simulink model "speedgoat_test_SN5659_R2021b"  (R2021b)
settings: Solver=FixedStepDiscrete  StartTime=0.0  StopTime=inf  RelTol=1e-3
PreLoadFcn:
  | Ts_IO107 = 0.001;
  | Ts_IO107 = 0.001;
  | Ts_IO133 = 0.001
  | 
  | Ts_IO204 = 0.001;
  | 
  | 
  | Ts_IO503 = 0.01;
  | 
  | ts_IO612 = 1e-3;
  | Ts_IO682 = 0.005;
  | Ts_IO941 = 0.01;
InitFcn:
  | Ts_IO107 = 0.001;
  | Ts_IO107 = 0.001;
  | Ts_IO133 = 0.001
  | 
  | Ts_IO204 = 0.001;
  | 
  | 
  | Ts_IO503 = 0.01;
  | 
  | ts_IO612 = 1e-3;
  | Ts_IO682 = 0.005;
  | Ts_IO941 = 0.01;
StopFcn:
  | if isfile(['sdi_view_',bdroot,'.mldatx'])
  |  Simulink.sdi.clearPreferences();
  |  Simulink.sdi.view();
  |  pause(3);
  |  Simulink.sdi.loadView(['sdi_view_',bdroot,]);
  | end
undefined symbols (not defined in the file): C, IO682, standard
libraries: speedgoatlib_IO682 x161, simulink x49, slrealtimeseriallib x16, canmsglib x12, speedgoatlib_serial x9, speedgoatlib_IO612 x9, speedgoatlib_IO133 x5, speedgoatlib_IO107 x4, speedgoatlib_IO204 x3, speedgoatlib_IO421 x3, speedgoatlib_PIL x1
(part 3 of 4)

== system speedgoat_test_SN5659_R2021b/IO682/Encode Channel 3 ==
  Constant : Constant  Value=150.159  SampleTime=Ts_IO682
  Counter Limited : simulink/Sources/Counter Limited  uplimit=300  tsamp=Ts_IO682
  Data Type Conversion : DataTypeConversion
  Encode 1 : speedgoatlib_IO682/Encode v2   parMode=Message Sequence  parLabel=100  parDataType=[1]  parResolution=[1024]  parBits=[10]  parSdi=[2]  parSsm=[3]  parCustomDataType=Raw  parDataLSB=9  parDataMSB=31  parBitPosition=[9, 31]  parScaleBNR=1  parExponent=8  parMantissa=14  parEnSSM=off
      settings: SourceProductName=Simulink Real-Time: Speedgoat I/O Blockset
  Encode 2 : speedgoatlib_IO682/Encode v2   parMode=Message Sequence  parLabel=101  parDataType=[2]  parResolution=[.1]  parBits=[0]  parSdi=[2]  parSsm=[0]  parCustomDataType=Raw  parDataLSB=9  parDataMSB=31  parBitPosition=[9, 31]  parScaleBNR=1  parExponent=8  parMantissa=14  parEnSSM=off
      settings: SourceProductName=Simulink Real-Time: Speedgoat I/O Blockset
  Encode 3 : speedgoatlib_IO682/Encode v2   parMode=Message Sequence  parLabel=102  parDataType=[1]  parResolution=[65536]  parBits=[16]  parSdi=[2]  parSsm=[3]  parCustomDataType=Raw  parDataLSB=9  parDataMSB=31  parBitPosition=[9, 31]  parScaleBNR=1  parExponent=8  parMantissa=14  parEnSSM=off
      settings: SourceProductName=Simulink Real-Time: Speedgoat I/O Blockset
  Encode 4 : speedgoatlib_IO682/Encode v2   parMode=Message Sequence  parLabel=103  parDataType=[0]  parResolution=[1]  parBits=[0]  parSdi=[0]  parSsm=[0]  parCustomDataType=Raw  parDataLSB=9  parDataMSB=31  parBitPosition=[9, 31]  parScaleBNR=1  parExponent=8  parMantissa=14  parEnSSM=off
      settings: SourceProductName=Simulink Real-Time: Speedgoat I/O Blockset
  Mux1 : Mux
  Prepare RAW value : Subsystem
  Random number : RandomNumber  Mean=150  Variance=10  SampleTime=Ts_IO682
  Sine wave : Sin  Amplitude=10000  Bias=13000  Frequency=2*pi*0.01  SampleTime=Ts_IO682
  Out1 : Outport
  wires:
  Encode 4/1 -> Mux1/4
  Mux1/1 -> Out1/1
  Counter Limited/1 -> Data Type Conversion/1
  Sine wave/1 -> Encode 3/1
  Encode 3/1 -> Mux1/3
  Encode 1/1 -> Mux1/1
  Random number/1 -> Encode 1/1
  Encode 2/1 -> Mux1/2
  Prepare RAW value/1(Out1) -> Encode 4/1
  Constant/1 -> Prepare RAW value/1(In1)
  Data Type Conversion/1 -> Encode 2/1

== system speedgoat_test_SN5659_R2021b/IO682/Encode Channel 4 ==
  Constant : Constant  Value=200.159  SampleTime=Ts_IO682
  Counter Limited : simulink/Sources/Counter Limited  uplimit=400  tsamp=Ts_IO682
  Data Type Conversion : DataTypeConversion
  Encode 1 : speedgoatlib_IO682/Encode v2   parMode=Message Sequence  parLabel=100  parDataType=[1]  parResolution=[1024]  parBits=[10]  parSdi=[2]  parSsm=[3]  parCustomDataType=Raw  parDataLSB=9  parDataMSB=31  parBitPosition=[9, 31]  parScaleBNR=1  parExponent=8  parMantissa=14  parEnSSM=off
      settings: SourceProductName=Simulink Real-Time: Speedgoat I/O Blockset
  Encode 2 : speedgoatlib_IO682/Encode v2   parMode=Message Sequence  parLabel=101  parDataType=[2]  parResolution=[.1]  parBits=[0]  parSdi=[2]  parSsm=[0]  parCustomDataType=Raw  parDataLSB=9  parDataMSB=31  parBitPosition=[9, 31]  parScaleBNR=1  parExponent=8  parMantissa=14  parEnSSM=off
      settings: SourceProductName=Simulink Real-Time: Speedgoat I/O Blockset
  Encode 3 : speedgoatlib_IO682/Encode v2   parMode=Message Sequence  parLabel=102  parDataType=[1]  parResolution=[65536]  parBits=[16]  parSdi=[2]  parSsm=[3]  parCustomDataType=Raw  parDataLSB=9  parDataMSB=31  parBitPosition=[9, 31]  parScaleBNR=1  parExponent=8  parMantissa=14  parEnSSM=off
      settings: SourceProductName=Simulink Real-Time: Speedgoat I/O Blockset
  Encode 4 : speedgoatlib_IO682/Encode v2   parMode=Message Sequence  parLabel=103  parDataType=[0]  parResolution=[1]  parBits=[0]  parSdi=[0]  parSsm=[0]  parCustomDataType=Raw  parDataLSB=9  parDataMSB=31  parBitPosition=[9, 31]  parScaleBNR=1  parExponent=8  parMantissa=14  parEnSSM=off
      settings: SourceProductName=Simulink Real-Time: Speedgoat I/O Blockset
  Mux1 : Mux
  Prepare RAW value : Subsystem
  Random number : RandomNumber  Mean=200  Variance=10  SampleTime=Ts_IO682
  Sine wave : Sin  Amplitude=10000  Bias=14000  Frequency=2*pi*0.01  SampleTime=Ts_IO682
  Out1 : Outport
  wires:
  Encode 4/1 -> Mux1/4
  Mux1/1 -> Out1/1
  Counter Limited/1 -> Data Type Conversion/1
  Sine wave/1 -> Encode 3/1
  Encode 3/1 -> Mux1/3
  Encode 1/1 -> Mux1/1
  Random number/1 -> Encode 1/1
  Encode 2/1 -> Mux1/2
  Prepare RAW value/1(Out1) -> Encode 4/1
  Constant/1 -> Prepare RAW value/1(In1)
  Data Type Conversion/1 -> Encode 2/1

== system speedgoat_test_SN5659_R2021b/IO682/Encode Channel 5 ==
  note: Encode block definitions:
      | 1. Label 100, BNR, Scale 1024, 10 bits, SDI 2, SSM 3
      | 2. Label 101, BCD, Resolution 0.1, SDI 2, SSM from sign of input
      | 3. Label 102, BNR, Scale 65536, 16 bits, SDI 2, SSM 3
      | 4. Label 103, RAW, Resolution/Scale, SDI and SSM aren't taken
      |         from the Encode block mask, but leave placeholders in the arrays.
      |         These values are inserted into the RAW value in the Prepare
      |         RAW value subsystem.  Label is also inserted manually.
  Constant : Constant  Value=250.159  SampleTime=Ts_IO682
  Counter Limited : simulink/Sources/Counter Limited  uplimit=500  tsamp=Ts_IO682
  Data Type Conversion : DataTypeConversion
  Encode 1 : speedgoatlib_IO682/Encode v2   parMode=Message Sequence  parLabel=100  parDataType=[1]  parResolution=[1024]  parBits=[10]  parSdi=[2]  parSsm=[3]  parCustomDataType=Raw  parDataLSB=9  parDataMSB=31  parBitPosition=[9, 31]  parScaleBNR=1  parExponent=8  parMantissa=14  parEnSSM=off
      settings: SourceProductName=Simulink Real-Time: Speedgoat I/O Blockset
  Encode 2 : speedgoatlib_IO682/Encode v2   parMode=Message Sequence  parLabel=103  parDataType=[0]  parResolution=[1024]  parBits=[0]  parSdi=[0]  parSsm=[0]  parCustomDataType=Raw  parDataLSB=9  parDataMSB=31  parBitPosition=[9, 31]  parScaleBNR=1  parExponent=8  parMantissa=14  parEnSSM=off
      settings: SourceProductName=Simulink Real-Time: Speedgoat I/O Blockset
  Encode 3 : speedgoatlib_IO682/Encode v2   parMode=Message Sequence  parLabel=102  parDataType=[1]  parResolution=[65536]  parBits=[16]  parSdi=[2]  parSsm=[3]  parCustomDataType=Raw  parDataLSB=9  parDataMSB=31  parBitPosition=[9, 31]  parScaleBNR=1  parExponent=8  parMantissa=14  parEnSSM=off
      settings: SourceProductName=Simulink Real-Time: Speedgoat I/O Blockset
  Encode 5 : speedgoatlib_IO682/Encode v2   parMode=Message Sequence  parLabel=101  parDataType=[2]  parResolution=[.1]  parBits=[0]  parSdi=[2]  parSsm=[0]  parCustomDataType=Raw  parDataLSB=9  parDataMSB=31  parBitPosition=[9, 31]  parScaleBNR=1  parExponent=8  parMantissa=14  parEnSSM=off
      settings: SourceProductName=Simulink Real-Time: Speedgoat I/O Blockset
  Mux : Mux
  Prepare RAW value : Subsystem
  Random number : RandomNumber  Mean=250  Variance=10  SampleTime=Ts_IO682
  Sine wave : Sin  Amplitude=10000  Bias=15000  Frequency=2*pi*0.01  SampleTime=Ts_IO682
  Out1 : Outport
  wires:
  Mux/1 -> Out1/1
  Sine wave/1 -> Encode 3/1
  Encode 2/1 -> Mux/4
  Encode 3/1 -> Mux/3
  Encode 5/1 -> Mux/2
  Random number/1 -> Encode 1/1
  Encode 1/1 -> Mux/1
  Counter Limited/1 -> Data Type Conversion/1
  Prepare RAW value/1(Out1) -> Encode 2/1
  Constant/1 -> Prepare RAW value/1(In1)
  Data Type Conversion/1 -> Encode 5/1

== system speedgoat_test_SN5659_R2021b/IO682/Encode Channel 6 ==
  Constant : Constant  Value=300.159  SampleTime=Ts_IO682
  Counter Limited : simulink/Sources/Counter Limited  uplimit=600  tsamp=Ts_IO682
  Data Type Conversion : DataTypeConversion
  Encode 1 : speedgoatlib_IO682/Encode v2   parMode=Message Sequence  parLabel=100  parDataType=[1]  parResolution=[1024]  parBits=[10]  parSdi=[2]  parSsm=[3]  parCustomDataType=Raw  parDataLSB=9  parDataMSB=31  parBitPosition=[9, 31]  parScaleBNR=1  parExponent=8  parMantissa=14  parEnSSM=off
      settings: SourceProductName=Simulink Real-Time: Speedgoat I/O Blockset
  Encode 2 : speedgoatlib_IO682/Encode v2   parMode=Message Sequence  parLabel=101  parDataType=[2]  parResolution=[.1]  parBits=[0]  parSdi=[2]  parSsm=[0]  parCustomDataType=Raw  parDataLSB=9  parDataMSB=31  parBitPosition=[9, 31]  parScaleBNR=1  parExponent=8  parMantissa=14  parEnSSM=off
      settings: SourceProductName=Simulink Real-Time: Speedgoat I/O Blockset
  Encode 3 : speedgoatlib_IO682/Encode v2   parMode=Message Sequence  parLabel=102  parDataType=[1]  parResolution=[65536]  parBits=[16]  parSdi=[2]  parSsm=[3]  parCustomDataType=Raw  parDataLSB=9  parDataMSB=31  parBitPosition=[9, 31]  parScaleBNR=1  parExponent=8  parMantissa=14  parEnSSM=off
      settings: SourceProductName=Simulink Real-Time: Speedgoat I/O Blockset
  Encode 4 : speedgoatlib_IO682/Encode v2   parMode=Message Sequence  parLabel=103  parDataType=[0]  parResolution=[1]  parBits=[0]  parSdi=[0]  parSsm=[0]  parCustomDataType=Raw  parDataLSB=9  parDataMSB=31  parBitPosition=[9, 31]  parScaleBNR=1  parExponent=8  parMantissa=14  parEnSSM=off
      settings: SourceProductName=Simulink Real-Time: Speedgoat I/O Blockset
  Mux1 : Mux
  Prepare RAW value : Subsystem
  Random number : RandomNumber  Mean=300  Variance=10  SampleTime=Ts_IO682
  Sine wave : Sin  Amplitude=10000  Bias=16000  Frequency=2*pi*0.01  SampleTime=Ts_IO682
  Out1 : Outport
  wires:
  Encode 2/1 -> Mux1/2
  Prepare RAW value/1(Out1) -> Encode 4/1
  Encode 3/1 -> Mux1/3
  Encode 1/1 -> Mux1/1
  Constant/1 -> Prepare RAW value/1(In1)
  Sine wave/1 -> Encode 3/1
  Random number/1 -> Encode 1/1
  Mux1/1 -> Out1/1
  Counter Limited/1 -> Data Type Conversion/1
  Encode 4/1 -> Mux1/4
  Data Type Conversion/1 -> Encode 2/1

== system speedgoat_test_SN5659_R2021b/IO682/Encode Channel 7 ==
  Constant : Constant  Value=350.159  SampleTime=Ts_IO682
  Counter Limited : simulink/Sources/Counter Limited  uplimit=700  tsamp=Ts_IO682
  Data Type Conversion : DataTypeConversion
  Encode 1 : speedgoatlib_IO682/Encode v2   parMode=Message Sequence  parLabel=100  parDataType=[1]  parResolution=[1024]  parBits=[10]  parSdi=[2]  parSsm=[3]  parCustomDataType=Raw  parDataLSB=9  parDataMSB=31  parBitPosition=[9, 31]  parScaleBNR=1  parExponent=8  parMantissa=14  parEnSSM=off
      settings: SourceProductName=Simulink Real-Time: Speedgoat I/O Blockset
  Encode 2 : speedgoatlib_IO682/Encode v2   parMode=Message Sequence  parLabel=101  parDataType=[2]  parResolution=[.1]  parBits=[0]  parSdi=[2]  parSsm=[0]  parCustomDataType=Raw  parDataLSB=9  parDataMSB=31  parBitPosition=[9, 31]  parScaleBNR=1  parExponent=8  parMantissa=14  parEnSSM=off
      settings: SourceProductName=Simulink Real-Time: Speedgoat I/O Blockset
  Encode 3 : speedgoatlib_IO682/Encode v2   parMode=Message Sequence  parLabel=102  parDataType=[1]  parResolution=[65536]  parBits=[16]  parSdi=[2]  parSsm=[3]  parCustomDataType=Raw  parDataLSB=9  parDataMSB=31  parBitPosition=[9, 31]  parScaleBNR=1  parExponent=8  parMantissa=14  parEnSSM=off
      settings: SourceProductName=Simulink Real-Time: Speedgoat I/O Blockset
  Encode 4 : speedgoatlib_IO682/Encode v2   parMode=Message Sequence  parLabel=103  parDataType=[0]  parResolution=[1]  parBits=[0]  parSdi=[0]  parSsm=[0]  parCustomDataType=Raw  parDataLSB=9  parDataMSB=31  parBitPosition=[9, 31]  parScaleBNR=1  parExponent=8  parMantissa=14  parEnSSM=off
      settings: SourceProductName=Simulink Real-Time: Speedgoat I/O Blockset
  Mux1 : Mux
  Prepare RAW value : Subsystem
  Random number : RandomNumber  Mean=350  Variance=10  SampleTime=Ts_IO682
  Sine wave : Sin  Amplitude=10000  Bias=17000  Frequency=2*pi*0.01  SampleTime=Ts_IO682
  Out1 : Outport
  wires:
  Encode 4/1 -> Mux1/4
  Mux1/1 -> Out1/1
  Counter Limited/1 -> Data Type Conversion/1
  Sine wave/1 -> Encode 3/1
  Encode 3/1 -> Mux1/3
  Encode 1/1 -> Mux1/1
  Random number/1 -> Encode 1/1
  Encode 2/1 -> Mux1/2
  Prepare RAW value/1(Out1) -> Encode 4/1
  Constant/1 -> Prepare RAW value/1(In1)
  Data Type Conversion/1 -> Encode 2/1

== system speedgoat_test_SN5659_R2021b/IO682/Encode Channel 8 ==
  Constant : Constant  Value=400.159  SampleTime=Ts_IO682
  Counter Limited : simulink/Sources/Counter Limited  uplimit=800  tsamp=Ts_IO682
  Data Type Conversion : DataTypeConversion
  Encode 1 : speedgoatlib_IO682/Encode v2   parMode=Message Sequence  parLabel=100  parDataType=[1]  parResolution=[1024]  parBits=[10]  parSdi=[2]  parSsm=[3]  parCustomDataType=Raw  parDataLSB=9  parDataMSB=31  parBitPosition=[9, 31]  parScaleBNR=1  parExponent=8  parMantissa=14  parEnSSM=off
      settings: SourceProductName=Simulink Real-Time: Speedgoat I/O Blockset
  Encode 2 : speedgoatlib_IO682/Encode v2   parMode=Message Sequence  parLabel=101  parDataType=[2]  parResolution=[.1]  parBits=[0]  parSdi=[2]  parSsm=[0]  parCustomDataType=Raw  parDataLSB=9  parDataMSB=31  parBitPosition=[9, 31]  parScaleBNR=1  parExponent=8  parMantissa=14  parEnSSM=off
      settings: SourceProductName=Simulink Real-Time: Speedgoat I/O Blockset
  Encode 3 : speedgoatlib_IO682/Encode v2   parMode=Message Sequence  parLabel=102  parDataType=[1]  parResolution=[65536]  parBits=[16]  parSdi=[2]  parSsm=[3]  parCustomDataType=Raw  parDataLSB=9  parDataMSB=31  parBitPosition=[9, 31]  parScaleBNR=1  parExponent=8  parMantissa=14  parEnSSM=off
      settings: SourceProductName=Simulink Real-Time: Speedgoat I/O Blockset
  Encode 4 : speedgoatlib_IO682/Encode v2   parMode=Message Sequence  parLabel=103  parDataType=[0]  parResolution=[1]  parBits=[0]  parSdi=[0]  parSsm=[0]  parCustomDataType=Raw  parDataLSB=9  parDataMSB=31  parBitPosition=[9, 31]  parScaleBNR=1  parExponent=8  parMantissa=14  parEnSSM=off
      settings: SourceProductName=Simulink Real-Time: Speedgoat I/O Blockset
  Mux1 : Mux
  Prepare RAW value : Subsystem
  Random number : RandomNumber  Mean=400  Variance=10  SampleTime=Ts_IO682
  Sine wave : Sin  Amplitude=10000  Bias=18000  Frequency=2*pi*0.01  SampleTime=Ts_IO682
  Out1 : Outport
  wires:
  Encode 4/1 -> Mux1/4
  Mux1/1 -> Out1/1
  Counter Limited/1 -> Data Type Conversion/1
  Sine wave/1 -> Encode 3/1
  Encode 3/1 -> Mux1/3
  Encode 1/1 -> Mux1/1
  Random number/1 -> Encode 1/1
  Encode 2/1 -> Mux1/2
  Prepare RAW value/1(Out1) -> Encode 4/1
  Constant/1 -> Prepare RAW value/1(In1)
  Data Type Conversion/1 -> Encode 2/1

== system speedgoat_test_SN5659_R2021b/IO682/Encode Channel 9 ==
  note: Encode block definitions:
      | 1. Label 100, BNR, Scale 1024, 10 bits, SDI 2, SSM 3
      | 2. Label 101, BCD, Resolution 0.1, SDI 2, SSM from sign of input
      | 3. Label 102, BNR, Scale 65536, 16 bits, SDI 2, SSM 3
      | 4. Label 103, RAW, Resolution/Scale, SDI and SSM aren't taken
      |         from the Encode block mask, but leave placeholders in the arrays.
      |         These values are inserted into the RAW value in the Prepare
      |         RAW value subsystem.  Label is also inserted manually.
  Constant : Constant  Value=450.159  SampleTime=Ts_IO682
  Counter Limited : simulink/Sources/Counter Limited  uplimit=900  tsamp=Ts_IO682
  Data Type Conversion : DataTypeConversion
  Encode 1 : speedgoatlib_IO682/Encode v2   parMode=Message Sequence  parLabel=100  parDataType=[1]  parResolution=[1024]  parBits=[10]  parSdi=[2]  parSsm=[3]  parCustomDataType=Raw  parDataLSB=9  parDataMSB=31  parBitPosition=[9, 31]  parScaleBNR=1  parExponent=8  parMantissa=14  parEnSSM=off
      settings: SourceProductName=Simulink Real-Time: Speedgoat I/O Blockset
  Encode 2 : speedgoatlib_IO682/Encode v2   parMode=Message Sequence  parLabel=103  parDataType=[0]  parResolution=[1024]  parBits=[0]  parSdi=[0]  parSsm=[0]  parCustomDataType=Raw  parDataLSB=9  parDataMSB=31  parBitPosition=[9, 31]  parScaleBNR=1  parExponent=8  parMantissa=14  parEnSSM=off
      settings: SourceProductName=Simulink Real-Time: Speedgoat I/O Blockset
  Encode 3 : speedgoatlib_IO682/Encode v2   parMode=Message Sequence  parLabel=102  parDataType=[1]  parResolution=[65536]  parBits=[16]  parSdi=[2]  parSsm=[3]  parCustomDataType=Raw  parDataLSB=9  parDataMSB=31  parBitPosition=[9, 31]  parScaleBNR=1  parExponent=8  parMantissa=14  parEnSSM=off
      settings: SourceProductName=Simulink Real-Time: Speedgoat I/O Blockset
  Encode 5 : speedgoatlib_IO682/Encode v2   parMode=Message Sequence  parLabel=101  parDataType=[2]  parResolution=[.1]  parBits=[0]  parSdi=[2]  parSsm=[0]  parCustomDataType=Raw  parDataLSB=9  parDataMSB=31  parBitPosition=[9, 31]  parScaleBNR=1  parExponent=8  parMantissa=14  parEnSSM=off
      settings: SourceProductName=Simulink Real-Time: Speedgoat I/O Blockset
  Mux : Mux
  Prepare RAW value : Subsystem
  Random number : RandomNumber  Mean=450  Variance=10  SampleTime=Ts_IO682
  Sine wave : Sin  Amplitude=10000  Bias=19000  Frequency=2*pi*0.01  SampleTime=Ts_IO682
  Out1 : Outport
  wires:
  Mux/1 -> Out1/1
  Sine wave/1 -> Encode 3/1
  Encode 2/1 -> Mux/4
  Encode 3/1 -> Mux/3
  Encode 5/1 -> Mux/2
  Random number/1 -> Encode 1/1
  Encode 1/1 -> Mux/1
  Counter Limited/1 -> Data Type Conversion/1
  Prepare RAW value/1(Out1) -> Encode 2/1
  Constant/1 -> Prepare RAW value/1(In1)
  Data Type Conversion/1 -> Encode 5/1

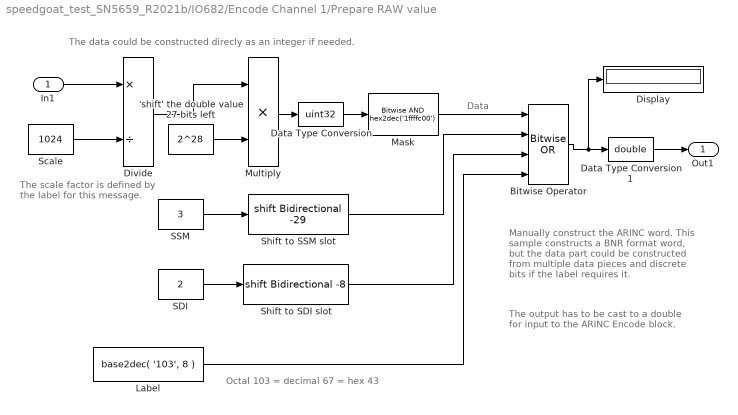
== system speedgoat_test_SN5659_R2021b/IO682/Encode Channel 1/Prepare RAW value ==
  note: The scale factor is
      | defined by the label
      | for this message.
  note: Manually construct the ARINC word.
      | This sample constructs a BNR format
      | word, but the data part could be
      | constructed from multiple data pieces
      | and discrete bits if the label requires it.
  note: Data
  note: The output has to be cast to a double
      | for input to the ARINC Encode block.
  note: The data could be constructed direcly as an integer if needed.
  note: Octal 103 = decimal 67 = hex 43
  In1 : Inport
  'shift' the double value 27 bits left : Constant  Value=2^28  OutDataTypeStr=double
  Bitwise Operator : simulink/Logic and Bit Operations/Bitwise Operator  logicop=OR  UseBitMask=off  NumInputPorts=4  BitMask=bin2dec('11011001')  BitMaskRealWorld=Stored Integer
  Data Type Conversion : DataTypeConversion  OutDataTypeStr=uint32
  Data Type Conversion1 : DataTypeConversion  OutDataTypeStr=double
  Display : Display
      settings: Format=hex (Stored Integer)
  Divide : Product  Inputs=*/
  Label : Constant  Value=base2dec( '103', 8 )  OutDataTypeStr=uint32
  "Mask " : simulink/Logic and Bit Operations/Bitwise Operator  logicop=AND  UseBitMask=on  BitMask=hex2dec('1ffffc00')  BitMaskRealWorld=Stored Integer
  Multiply : Product  Inputs=**
  SDI : Constant  Value=2  OutDataTypeStr=uint32
  SSM : Constant  Value=3  OutDataTypeStr=uint32
  Scale : Constant  Value=1024  OutDataTypeStr=double
  Shift to SDI slot : ArithShift  BitShiftNumber=-8
  Shift to SSM slot : ArithShift  BitShiftNumber=-29
  Out1 : Outport
  wires:
  In1/1 -> Divide/1
  Scale/1 -> Divide/2
  'shift' the double value 27 bits left/1 -> Multiply/2
  Divide/1 -> Multiply/1
  Multiply/1 -> Data Type Conversion/1
  Data Type Conversion/1 -> "Mask "/1
  "Mask "/1 -> Bitwise Operator/1
  SSM/1 -> Shift to SSM slot/1
  SDI/1 -> Shift to SDI slot/1
  Shift to SSM slot/1 -> Bitwise Operator/2
  Shift to SDI slot/1 -> Bitwise Operator/3
  Label/1 -> Bitwise Operator/4
  Bitwise Operator/1 -> Data Type Conversion1/1, Display/1
  Data Type Conversion1/1 -> Out1/1

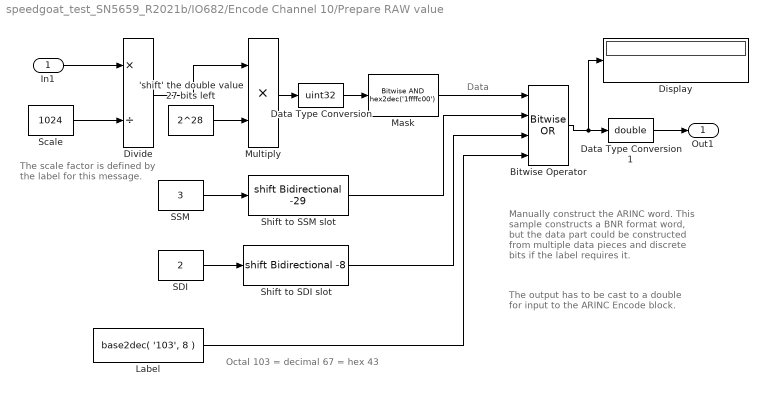
== system speedgoat_test_SN5659_R2021b/IO682/Encode Channel 10/Prepare RAW value ==
  note: Octal 103 = decimal 67 = hex 43
  note: The output has to be cast to a double
      | for input to the ARINC Encode block.
  note: Data
  note: Manually construct the ARINC word.
      | This sample constructs a BNR format
      | word, but the data part could be
      | constructed from multiple data pieces
      | and discrete bits if the label requires it.
  note: The scale factor is
      | defined by the label
      | for this message.
  In1 : Inport
  'shift' the double value 27 bits left : Constant  Value=2^28  OutDataTypeStr=double
  Bitwise Operator : simulink/Logic and Bit Operations/Bitwise Operator  logicop=OR  UseBitMask=off  NumInputPorts=4  BitMask=bin2dec('11011001')  BitMaskRealWorld=Stored Integer
  Data Type Conversion : DataTypeConversion  OutDataTypeStr=uint32
  Data Type Conversion1 : DataTypeConversion  OutDataTypeStr=double
  Display : Display
      settings: Format=hex (Stored Integer)
  Divide : Product  Inputs=*/
  Label : Constant  Value=base2dec( '103', 8 )  OutDataTypeStr=uint32
  "Mask " : simulink/Logic and Bit Operations/Bitwise Operator  logicop=AND  UseBitMask=on  BitMask=hex2dec('1ffffc00')  BitMaskRealWorld=Stored Integer
  Multiply : Product  Inputs=**
  SDI : Constant  Value=2  OutDataTypeStr=uint32
  SSM : Constant  Value=3  OutDataTypeStr=uint32
  Scale : Constant  Value=1024  OutDataTypeStr=double
  Shift to SDI slot : ArithShift  BitShiftNumber=-8
  Shift to SSM slot : ArithShift  BitShiftNumber=-29
  Out1 : Outport
  wires:
  Data Type Conversion1/1 -> Out1/1
  Bitwise Operator/1 -> Display/1, Data Type Conversion1/1
  Label/1 -> Bitwise Operator/4
  Shift to SDI slot/1 -> Bitwise Operator/3
  Shift to SSM slot/1 -> Bitwise Operator/2
  SDI/1 -> Shift to SDI slot/1
  SSM/1 -> Shift to SSM slot/1
  "Mask "/1 -> Bitwise Operator/1
  Data Type Conversion/1 -> "Mask "/1
  Multiply/1 -> Data Type Conversion/1
  Divide/1 -> Multiply/1
  'shift' the double value 27 bits left/1 -> Multiply/2
  Scale/1 -> Divide/2
  In1/1 -> Divide/1

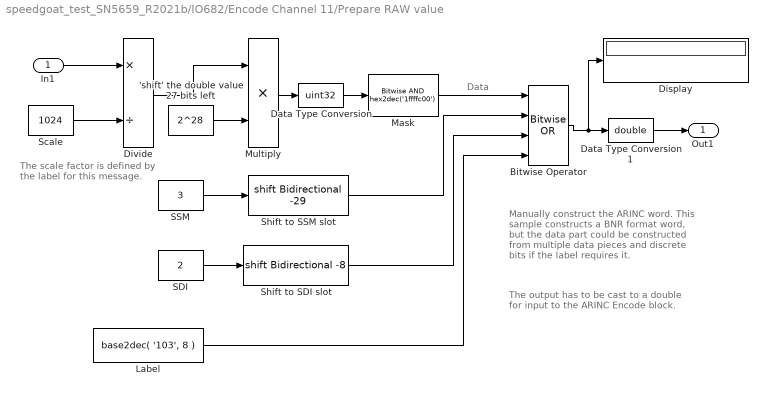
== system speedgoat_test_SN5659_R2021b/IO682/Encode Channel 11/Prepare RAW value ==
  note: The scale factor is
      | defined by the label
      | for this message.
  note: Manually construct the ARINC word.
      | This sample constructs a BNR format
      | word, but the data part could be
      | constructed from multiple data pieces
      | and discrete bits if the label requires it.
  note: Data
  note: The output has to be cast to a double
      | for input to the ARINC Encode block.
  In1 : Inport
  'shift' the double value 27 bits left : Constant  Value=2^28  OutDataTypeStr=double
  Bitwise Operator : simulink/Logic and Bit Operations/Bitwise Operator  logicop=OR  UseBitMask=off  NumInputPorts=4  BitMask=bin2dec('11011001')  BitMaskRealWorld=Stored Integer
  Data Type Conversion : DataTypeConversion  OutDataTypeStr=uint32
  Data Type Conversion1 : DataTypeConversion  OutDataTypeStr=double
  Display : Display
      settings: Format=hex (Stored Integer)
  Divide : Product  Inputs=*/
  Label : Constant  Value=base2dec( '103', 8 )  OutDataTypeStr=uint32
  "Mask " : simulink/Logic and Bit Operations/Bitwise Operator  logicop=AND  UseBitMask=on  BitMask=hex2dec('1ffffc00')  BitMaskRealWorld=Stored Integer
  Multiply : Product  Inputs=**
  SDI : Constant  Value=2  OutDataTypeStr=uint32
  SSM : Constant  Value=3  OutDataTypeStr=uint32
  Scale : Constant  Value=1024  OutDataTypeStr=double
  Shift to SDI slot : ArithShift  BitShiftNumber=-8
  Shift to SSM slot : ArithShift  BitShiftNumber=-29
  Out1 : Outport
  wires:
  In1/1 -> Divide/1
  Scale/1 -> Divide/2
  'shift' the double value 27 bits left/1 -> Multiply/2
  Divide/1 -> Multiply/1
  Multiply/1 -> Data Type Conversion/1
  Data Type Conversion/1 -> "Mask "/1
  "Mask "/1 -> Bitwise Operator/1
  SSM/1 -> Shift to SSM slot/1
  SDI/1 -> Shift to SDI slot/1
  Shift to SSM slot/1 -> Bitwise Operator/2
  Shift to SDI slot/1 -> Bitwise Operator/3
  Label/1 -> Bitwise Operator/4
  Bitwise Operator/1 -> Data Type Conversion1/1, Display/1
  Data Type Conversion1/1 -> Out1/1

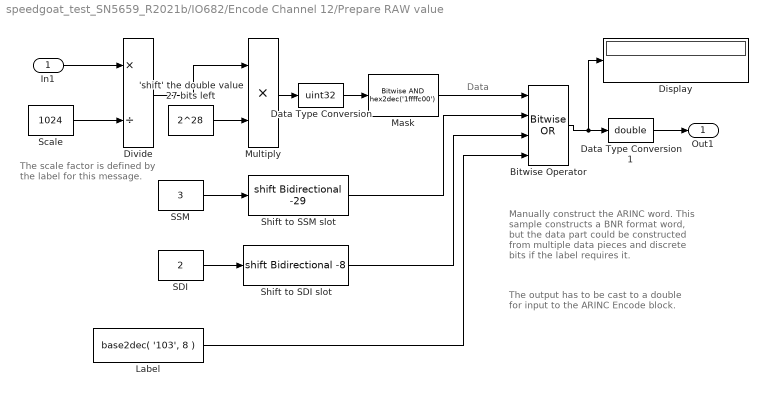
== system speedgoat_test_SN5659_R2021b/IO682/Encode Channel 12/Prepare RAW value ==
  note: The output has to be cast to a double
      | for input to the ARINC Encode block.
  note: Data
  note: Manually construct the ARINC word.
      | This sample constructs a BNR format
      | word, but the data part could be
      | constructed from multiple data pieces
      | and discrete bits if the label requires it.
  note: The scale factor is
      | defined by the label
      | for this message.
  In1 : Inport
  'shift' the double value 27 bits left : Constant  Value=2^28  OutDataTypeStr=double
  Bitwise Operator : simulink/Logic and Bit Operations/Bitwise Operator  logicop=OR  UseBitMask=off  NumInputPorts=4  BitMask=bin2dec('11011001')  BitMaskRealWorld=Stored Integer
  Data Type Conversion : DataTypeConversion  OutDataTypeStr=uint32
  Data Type Conversion1 : DataTypeConversion  OutDataTypeStr=double
  Display : Display
      settings: Format=hex (Stored Integer)
  Divide : Product  Inputs=*/
  Label : Constant  Value=base2dec( '103', 8 )  OutDataTypeStr=uint32
  "Mask " : simulink/Logic and Bit Operations/Bitwise Operator  logicop=AND  UseBitMask=on  BitMask=hex2dec('1ffffc00')  BitMaskRealWorld=Stored Integer
  Multiply : Product  Inputs=**
  SDI : Constant  Value=2  OutDataTypeStr=uint32
  SSM : Constant  Value=3  OutDataTypeStr=uint32
  Scale : Constant  Value=1024  OutDataTypeStr=double
  Shift to SDI slot : ArithShift  BitShiftNumber=-8
  Shift to SSM slot : ArithShift  BitShiftNumber=-29
  Out1 : Outport
  wires:
  Data Type Conversion1/1 -> Out1/1
  Bitwise Operator/1 -> Display/1, Data Type Conversion1/1
  Label/1 -> Bitwise Operator/4
  Shift to SDI slot/1 -> Bitwise Operator/3
  Shift to SSM slot/1 -> Bitwise Operator/2
  SDI/1 -> Shift to SDI slot/1
  SSM/1 -> Shift to SSM slot/1
  "Mask "/1 -> Bitwise Operator/1
  Data Type Conversion/1 -> "Mask "/1
  Multiply/1 -> Data Type Conversion/1
  Divide/1 -> Multiply/1
  'shift' the double value 27 bits left/1 -> Multiply/2
  Scale/1 -> Divide/2
  In1/1 -> Divide/1

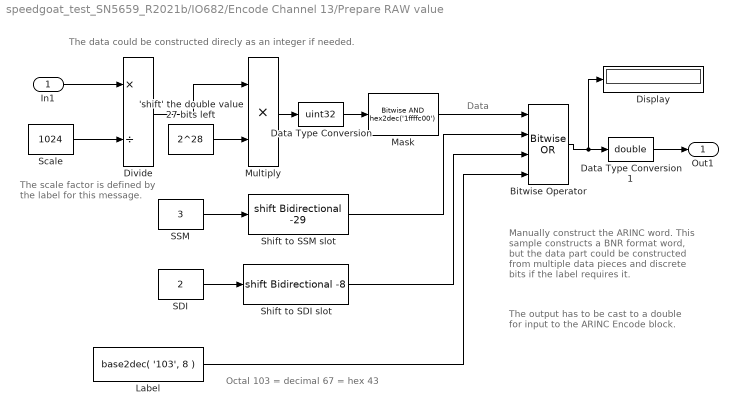
== system speedgoat_test_SN5659_R2021b/IO682/Encode Channel 13/Prepare RAW value ==
  note: The scale factor is
      | defined by the label
      | for this message.
  note: Manually construct the ARINC word.
      | This sample constructs a BNR format
      | word, but the data part could be
      | constructed from multiple data pieces
      | and discrete bits if the label requires it.
  note: Data
  note: The output has to be cast to a double
      | for input to the ARINC Encode block.
  note: The data could be constructed direcly as an integer if needed.
  note: Octal 103 = decimal 67 = hex 43
  In1 : Inport
  'shift' the double value 27 bits left : Constant  Value=2^28  OutDataTypeStr=double
  Bitwise Operator : simulink/Logic and Bit Operations/Bitwise Operator  logicop=OR  UseBitMask=off  NumInputPorts=4  BitMask=bin2dec('11011001')  BitMaskRealWorld=Stored Integer
  Data Type Conversion : DataTypeConversion  OutDataTypeStr=uint32
  Data Type Conversion1 : DataTypeConversion  OutDataTypeStr=double
  Display : Display
      settings: Format=hex (Stored Integer)
  Divide : Product  Inputs=*/
  Label : Constant  Value=base2dec( '103', 8 )  OutDataTypeStr=uint32
  "Mask " : simulink/Logic and Bit Operations/Bitwise Operator  logicop=AND  UseBitMask=on  BitMask=hex2dec('1ffffc00')  BitMaskRealWorld=Stored Integer
  Multiply : Product  Inputs=**
  SDI : Constant  Value=2  OutDataTypeStr=uint32
  SSM : Constant  Value=3  OutDataTypeStr=uint32
  Scale : Constant  Value=1024  OutDataTypeStr=double
  Shift to SDI slot : ArithShift  BitShiftNumber=-8
  Shift to SSM slot : ArithShift  BitShiftNumber=-29
  Out1 : Outport
  wires:
  In1/1 -> Divide/1
  Scale/1 -> Divide/2
  'shift' the double value 27 bits left/1 -> Multiply/2
  Divide/1 -> Multiply/1
  Multiply/1 -> Data Type Conversion/1
  Data Type Conversion/1 -> "Mask "/1
  "Mask "/1 -> Bitwise Operator/1
  SSM/1 -> Shift to SSM slot/1
  SDI/1 -> Shift to SDI slot/1
  Shift to SSM slot/1 -> Bitwise Operator/2
  Shift to SDI slot/1 -> Bitwise Operator/3
  Label/1 -> Bitwise Operator/4
  Bitwise Operator/1 -> Data Type Conversion1/1, Display/1
  Data Type Conversion1/1 -> Out1/1

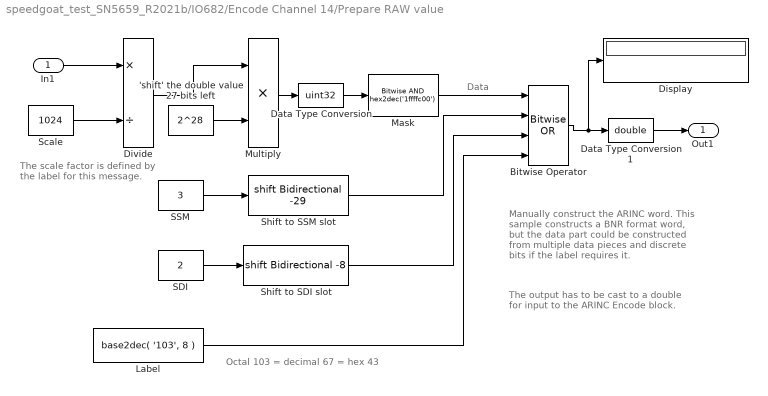
== system speedgoat_test_SN5659_R2021b/IO682/Encode Channel 14/Prepare RAW value ==
  note: Octal 103 = decimal 67 = hex 43
  note: The output has to be cast to a double
      | for input to the ARINC Encode block.
  note: Data
  note: Manually construct the ARINC word.
      | This sample constructs a BNR format
      | word, but the data part could be
      | constructed from multiple data pieces
      | and discrete bits if the label requires it.
  note: The scale factor is
      | defined by the label
      | for this message.
  In1 : Inport
  'shift' the double value 27 bits left : Constant  Value=2^28  OutDataTypeStr=double
  Bitwise Operator : simulink/Logic and Bit Operations/Bitwise Operator  logicop=OR  UseBitMask=off  NumInputPorts=4  BitMask=bin2dec('11011001')  BitMaskRealWorld=Stored Integer
  Data Type Conversion : DataTypeConversion  OutDataTypeStr=uint32
  Data Type Conversion1 : DataTypeConversion  OutDataTypeStr=double
  Display : Display
      settings: Format=hex (Stored Integer)
  Divide : Product  Inputs=*/
  Label : Constant  Value=base2dec( '103', 8 )  OutDataTypeStr=uint32
  "Mask " : simulink/Logic and Bit Operations/Bitwise Operator  logicop=AND  UseBitMask=on  BitMask=hex2dec('1ffffc00')  BitMaskRealWorld=Stored Integer
  Multiply : Product  Inputs=**
  SDI : Constant  Value=2  OutDataTypeStr=uint32
  SSM : Constant  Value=3  OutDataTypeStr=uint32
  Scale : Constant  Value=1024  OutDataTypeStr=double
  Shift to SDI slot : ArithShift  BitShiftNumber=-8
  Shift to SSM slot : ArithShift  BitShiftNumber=-29
  Out1 : Outport
  wires:
  Data Type Conversion1/1 -> Out1/1
  Bitwise Operator/1 -> Display/1, Data Type Conversion1/1
  Label/1 -> Bitwise Operator/4
  Shift to SDI slot/1 -> Bitwise Operator/3
  Shift to SSM slot/1 -> Bitwise Operator/2
  SDI/1 -> Shift to SDI slot/1
  SSM/1 -> Shift to SSM slot/1
  "Mask "/1 -> Bitwise Operator/1
  Data Type Conversion/1 -> "Mask "/1
  Multiply/1 -> Data Type Conversion/1
  Divide/1 -> Multiply/1
  'shift' the double value 27 bits left/1 -> Multiply/2
  Scale/1 -> Divide/2
  In1/1 -> Divide/1

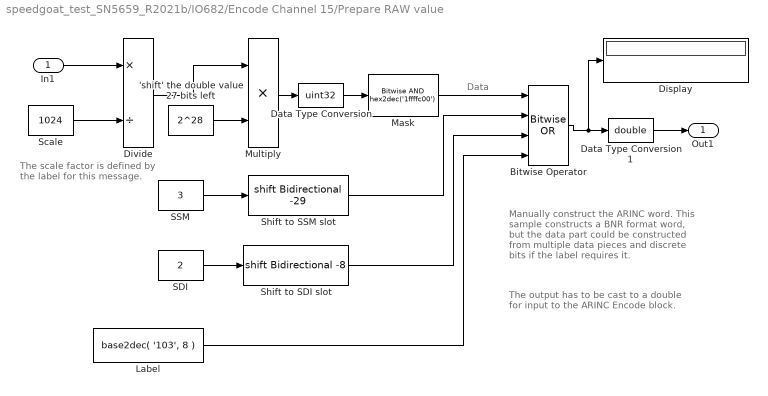
== system speedgoat_test_SN5659_R2021b/IO682/Encode Channel 15/Prepare RAW value ==
  note: The scale factor is
      | defined by the label
      | for this message.
  note: Manually construct the ARINC word.
      | This sample constructs a BNR format
      | word, but the data part could be
      | constructed from multiple data pieces
      | and discrete bits if the label requires it.
  note: Data
  note: The output has to be cast to a double
      | for input to the ARINC Encode block.
  In1 : Inport
  'shift' the double value 27 bits left : Constant  Value=2^28  OutDataTypeStr=double
  Bitwise Operator : simulink/Logic and Bit Operations/Bitwise Operator  logicop=OR  UseBitMask=off  NumInputPorts=4  BitMask=bin2dec('11011001')  BitMaskRealWorld=Stored Integer
  Data Type Conversion : DataTypeConversion  OutDataTypeStr=uint32
  Data Type Conversion1 : DataTypeConversion  OutDataTypeStr=double
  Display : Display
      settings: Format=hex (Stored Integer)
  Divide : Product  Inputs=*/
  Label : Constant  Value=base2dec( '103', 8 )  OutDataTypeStr=uint32
  "Mask " : simulink/Logic and Bit Operations/Bitwise Operator  logicop=AND  UseBitMask=on  BitMask=hex2dec('1ffffc00')  BitMaskRealWorld=Stored Integer
  Multiply : Product  Inputs=**
  SDI : Constant  Value=2  OutDataTypeStr=uint32
  SSM : Constant  Value=3  OutDataTypeStr=uint32
  Scale : Constant  Value=1024  OutDataTypeStr=double
  Shift to SDI slot : ArithShift  BitShiftNumber=-8
  Shift to SSM slot : ArithShift  BitShiftNumber=-29
  Out1 : Outport
  wires:
  In1/1 -> Divide/1
  Scale/1 -> Divide/2
  'shift' the double value 27 bits left/1 -> Multiply/2
  Divide/1 -> Multiply/1
  Multiply/1 -> Data Type Conversion/1
  Data Type Conversion/1 -> "Mask "/1
  "Mask "/1 -> Bitwise Operator/1
  SSM/1 -> Shift to SSM slot/1
  SDI/1 -> Shift to SDI slot/1
  Shift to SSM slot/1 -> Bitwise Operator/2
  Shift to SDI slot/1 -> Bitwise Operator/3
  Label/1 -> Bitwise Operator/4
  Bitwise Operator/1 -> Data Type Conversion1/1, Display/1
  Data Type Conversion1/1 -> Out1/1

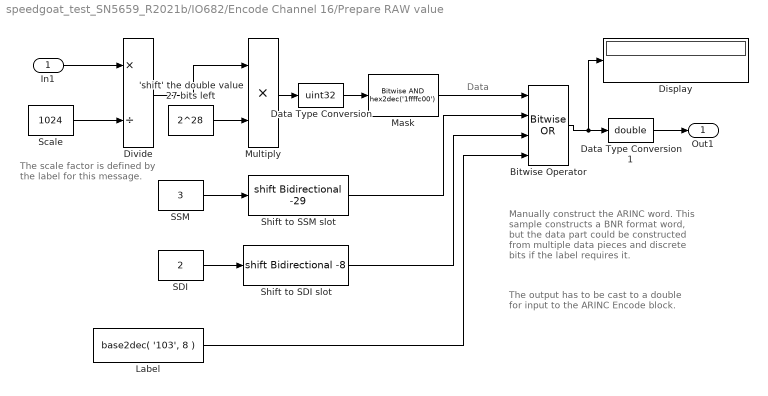
== system speedgoat_test_SN5659_R2021b/IO682/Encode Channel 16/Prepare RAW value ==
  note: The output has to be cast to a double
      | for input to the ARINC Encode block.
  note: Data
  note: Manually construct the ARINC word.
      | This sample constructs a BNR format
      | word, but the data part could be
      | constructed from multiple data pieces
      | and discrete bits if the label requires it.
  note: The scale factor is
      | defined by the label
      | for this message.
  In1 : Inport
  'shift' the double value 27 bits left : Constant  Value=2^28  OutDataTypeStr=double
  Bitwise Operator : simulink/Logic and Bit Operations/Bitwise Operator  logicop=OR  UseBitMask=off  NumInputPorts=4  BitMask=bin2dec('11011001')  BitMaskRealWorld=Stored Integer
  Data Type Conversion : DataTypeConversion  OutDataTypeStr=uint32
  Data Type Conversion1 : DataTypeConversion  OutDataTypeStr=double
  Display : Display
      settings: Format=hex (Stored Integer)
  Divide : Product  Inputs=*/
  Label : Constant  Value=base2dec( '103', 8 )  OutDataTypeStr=uint32
  "Mask " : simulink/Logic and Bit Operations/Bitwise Operator  logicop=AND  UseBitMask=on  BitMask=hex2dec('1ffffc00')  BitMaskRealWorld=Stored Integer
  Multiply : Product  Inputs=**
  SDI : Constant  Value=2  OutDataTypeStr=uint32
  SSM : Constant  Value=3  OutDataTypeStr=uint32
  Scale : Constant  Value=1024  OutDataTypeStr=double
  Shift to SDI slot : ArithShift  BitShiftNumber=-8
  Shift to SSM slot : ArithShift  BitShiftNumber=-29
  Out1 : Outport
  wires:
  Data Type Conversion1/1 -> Out1/1
  Bitwise Operator/1 -> Display/1, Data Type Conversion1/1
  Label/1 -> Bitwise Operator/4
  Shift to SDI slot/1 -> Bitwise Operator/3
  Shift to SSM slot/1 -> Bitwise Operator/2
  SDI/1 -> Shift to SDI slot/1
  SSM/1 -> Shift to SSM slot/1
  "Mask "/1 -> Bitwise Operator/1
  Data Type Conversion/1 -> "Mask "/1
  Multiply/1 -> Data Type Conversion/1
  Divide/1 -> Multiply/1
  'shift' the double value 27 bits left/1 -> Multiply/2
  Scale/1 -> Divide/2
  In1/1 -> Divide/1

== system speedgoat_test_SN5659_R2021b/IO682/Encode Channel 2/Prepare RAW value ==
  note: Octal 103 = decimal 67 = hex 43
  note: The output has to be cast to a double
      | for input to the ARINC Encode block.
  note: Data
  note: Manually construct the ARINC word.
      | This sample constructs a BNR format
      | word, but the data part could be
      | constructed from multiple data pieces
      | and discrete bits if the label requires it.
  note: The scale factor is
      | defined by the label
      | for this message.
  In1 : Inport
  'shift' the double value 27 bits left : Constant  Value=2^28  OutDataTypeStr=double
  Bitwise Operator : simulink/Logic and Bit Operations/Bitwise Operator  logicop=OR  UseBitMask=off  NumInputPorts=4  BitMask=bin2dec('11011001')  BitMaskRealWorld=Stored Integer
  Data Type Conversion : DataTypeConversion  OutDataTypeStr=uint32
  Data Type Conversion1 : DataTypeConversion  OutDataTypeStr=double
  Display : Display
      settings: Format=hex (Stored Integer)
  Divide : Product  Inputs=*/
  Label : Constant  Value=base2dec( '103', 8 )  OutDataTypeStr=uint32
  "Mask " : simulink/Logic and Bit Operations/Bitwise Operator  logicop=AND  UseBitMask=on  BitMask=hex2dec('1ffffc00')  BitMaskRealWorld=Stored Integer
  Multiply : Product  Inputs=**
  SDI : Constant  Value=2  OutDataTypeStr=uint32
  SSM : Constant  Value=3  OutDataTypeStr=uint32
  Scale : Constant  Value=1024  OutDataTypeStr=double
  Shift to SDI slot : ArithShift  BitShiftNumber=-8
  Shift to SSM slot : ArithShift  BitShiftNumber=-29
  Out1 : Outport
  wires:
  Data Type Conversion1/1 -> Out1/1
  Bitwise Operator/1 -> Display/1, Data Type Conversion1/1
  Label/1 -> Bitwise Operator/4
  Shift to SDI slot/1 -> Bitwise Operator/3
  Shift to SSM slot/1 -> Bitwise Operator/2
  SDI/1 -> Shift to SDI slot/1
  SSM/1 -> Shift to SSM slot/1
  "Mask "/1 -> Bitwise Operator/1
  Data Type Conversion/1 -> "Mask "/1
  Multiply/1 -> Data Type Conversion/1
  Divide/1 -> Multiply/1
  'shift' the double value 27 bits left/1 -> Multiply/2
  Scale/1 -> Divide/2
  In1/1 -> Divide/1

== system speedgoat_test_SN5659_R2021b/IO682/Encode Channel 3/Prepare RAW value ==
  note: The scale factor is
      | defined by the label
      | for this message.
  note: Manually construct the ARINC word.
      | This sample constructs a BNR format
      | word, but the data part could be
      | constructed from multiple data pieces
      | and discrete bits if the label requires it.
  note: Data
  note: The output has to be cast to a double
      | for input to the ARINC Encode block.
  In1 : Inport
  'shift' the double value 27 bits left : Constant  Value=2^28  OutDataTypeStr=double
  Bitwise Operator : simulink/Logic and Bit Operations/Bitwise Operator  logicop=OR  UseBitMask=off  NumInputPorts=4  BitMask=bin2dec('11011001')  BitMaskRealWorld=Stored Integer
  Data Type Conversion : DataTypeConversion  OutDataTypeStr=uint32
  Data Type Conversion1 : DataTypeConversion  OutDataTypeStr=double
  Display : Display
      settings: Format=hex (Stored Integer)
  Divide : Product  Inputs=*/
  Label : Constant  Value=base2dec( '103', 8 )  OutDataTypeStr=uint32
  "Mask " : simulink/Logic and Bit Operations/Bitwise Operator  logicop=AND  UseBitMask=on  BitMask=hex2dec('1ffffc00')  BitMaskRealWorld=Stored Integer
  Multiply : Product  Inputs=**
  SDI : Constant  Value=2  OutDataTypeStr=uint32
  SSM : Constant  Value=3  OutDataTypeStr=uint32
  Scale : Constant  Value=1024  OutDataTypeStr=double
  Shift to SDI slot : ArithShift  BitShiftNumber=-8
  Shift to SSM slot : ArithShift  BitShiftNumber=-29
  Out1 : Outport
  wires:
  In1/1 -> Divide/1
  Scale/1 -> Divide/2
  'shift' the double value 27 bits left/1 -> Multiply/2
  Divide/1 -> Multiply/1
  Multiply/1 -> Data Type Conversion/1
  Data Type Conversion/1 -> "Mask "/1
  "Mask "/1 -> Bitwise Operator/1
  SSM/1 -> Shift to SSM slot/1
  SDI/1 -> Shift to SDI slot/1
  Shift to SSM slot/1 -> Bitwise Operator/2
  Shift to SDI slot/1 -> Bitwise Operator/3
  Label/1 -> Bitwise Operator/4
  Bitwise Operator/1 -> Data Type Conversion1/1, Display/1
  Data Type Conversion1/1 -> Out1/1

== system speedgoat_test_SN5659_R2021b/IO682/Encode Channel 4/Prepare RAW value ==
  note: The output has to be cast to a double
      | for input to the ARINC Encode block.
  note: Data
  note: Manually construct the ARINC word.
      | This sample constructs a BNR format
      | word, but the data part could be
      | constructed from multiple data pieces
      | and discrete bits if the label requires it.
  note: The scale factor is
      | defined by the label
      | for this message.
  In1 : Inport
  'shift' the double value 27 bits left : Constant  Value=2^28  OutDataTypeStr=double
  Bitwise Operator : simulink/Logic and Bit Operations/Bitwise Operator  logicop=OR  UseBitMask=off  NumInputPorts=4  BitMask=bin2dec('11011001')  BitMaskRealWorld=Stored Integer
  Data Type Conversion : DataTypeConversion  OutDataTypeStr=uint32
  Data Type Conversion1 : DataTypeConversion  OutDataTypeStr=double
  Display : Display
      settings: Format=hex (Stored Integer)
  Divide : Product  Inputs=*/
  Label : Constant  Value=base2dec( '103', 8 )  OutDataTypeStr=uint32
  "Mask " : simulink/Logic and Bit Operations/Bitwise Operator  logicop=AND  UseBitMask=on  BitMask=hex2dec('1ffffc00')  BitMaskRealWorld=Stored Integer
  Multiply : Product  Inputs=**
  SDI : Constant  Value=2  OutDataTypeStr=uint32
  SSM : Constant  Value=3  OutDataTypeStr=uint32
  Scale : Constant  Value=1024  OutDataTypeStr=double
  Shift to SDI slot : ArithShift  BitShiftNumber=-8
  Shift to SSM slot : ArithShift  BitShiftNumber=-29
  Out1 : Outport
  wires:
  Data Type Conversion1/1 -> Out1/1
  Bitwise Operator/1 -> Display/1, Data Type Conversion1/1
  Label/1 -> Bitwise Operator/4
  Shift to SDI slot/1 -> Bitwise Operator/3
  Shift to SSM slot/1 -> Bitwise Operator/2
  SDI/1 -> Shift to SDI slot/1
  SSM/1 -> Shift to SSM slot/1
  "Mask "/1 -> Bitwise Operator/1
  Data Type Conversion/1 -> "Mask "/1
  Multiply/1 -> Data Type Conversion/1
  Divide/1 -> Multiply/1
  'shift' the double value 27 bits left/1 -> Multiply/2
  Scale/1 -> Divide/2
  In1/1 -> Divide/1

== system speedgoat_test_SN5659_R2021b/IO682/Encode Channel 5/Prepare RAW value ==
  note: The scale factor is
      | defined by the label
      | for this message.
  note: Manually construct the ARINC word.
      | This sample constructs a BNR format
      | word, but the data part could be
      | constructed from multiple data pieces
      | and discrete bits if the label requires it.
  note: Data
  note: The output has to be cast to a double
      | for input to the ARINC Encode block.
  note: The data could be constructed direcly as an integer if needed.
  note: Octal 103 = decimal 67 = hex 43
  In1 : Inport
  'shift' the double value 27 bits left : Constant  Value=2^28  OutDataTypeStr=double
  Bitwise Operator : simulink/Logic and Bit Operations/Bitwise Operator  logicop=OR  UseBitMask=off  NumInputPorts=4  BitMask=bin2dec('11011001')  BitMaskRealWorld=Stored Integer
  Data Type Conversion : DataTypeConversion  OutDataTypeStr=uint32
  Data Type Conversion1 : DataTypeConversion  OutDataTypeStr=double
  Display : Display
      settings: Format=hex (Stored Integer)
  Divide : Product  Inputs=*/
  Label : Constant  Value=base2dec( '103', 8 )  OutDataTypeStr=uint32
  "Mask " : simulink/Logic and Bit Operations/Bitwise Operator  logicop=AND  UseBitMask=on  BitMask=hex2dec('1ffffc00')  BitMaskRealWorld=Stored Integer
  Multiply : Product  Inputs=**
  SDI : Constant  Value=2  OutDataTypeStr=uint32
  SSM : Constant  Value=3  OutDataTypeStr=uint32
  Scale : Constant  Value=1024  OutDataTypeStr=double
  Shift to SDI slot : ArithShift  BitShiftNumber=-8
  Shift to SSM slot : ArithShift  BitShiftNumber=-29
  Out1 : Outport
  wires:
  In1/1 -> Divide/1
  Scale/1 -> Divide/2
  'shift' the double value 27 bits left/1 -> Multiply/2
  Divide/1 -> Multiply/1
  Multiply/1 -> Data Type Conversion/1
  Data Type Conversion/1 -> "Mask "/1
  "Mask "/1 -> Bitwise Operator/1
  SSM/1 -> Shift to SSM slot/1
  SDI/1 -> Shift to SDI slot/1
  Shift to SSM slot/1 -> Bitwise Operator/2
  Shift to SDI slot/1 -> Bitwise Operator/3
  Label/1 -> Bitwise Operator/4
  Bitwise Operator/1 -> Data Type Conversion1/1, Display/1
  Data Type Conversion1/1 -> Out1/1

== system speedgoat_test_SN5659_R2021b/IO682/Encode Channel 6/Prepare RAW value ==
  note: Octal 103 = decimal 67 = hex 43
  note: The output has to be cast to a double
      | for input to the ARINC Encode block.
  note: Data
  note: Manually construct the ARINC word.
      | This sample constructs a BNR format
      | word, but the data part could be
      | constructed from multiple data pieces
      | and discrete bits if the label requires it.
  note: The scale factor is
      | defined by the label
      | for this message.
  In1 : Inport
  'shift' the double value 27 bits left : Constant  Value=2^28  OutDataTypeStr=double
  Bitwise Operator : simulink/Logic and Bit Operations/Bitwise Operator  logicop=OR  UseBitMask=off  NumInputPorts=4  BitMask=bin2dec('11011001')  BitMaskRealWorld=Stored Integer
  Data Type Conversion : DataTypeConversion  OutDataTypeStr=uint32
  Data Type Conversion1 : DataTypeConversion  OutDataTypeStr=double
  Display : Display
      settings: Format=hex (Stored Integer)
  Divide : Product  Inputs=*/
  Label : Constant  Value=base2dec( '103', 8 )  OutDataTypeStr=uint32
  "Mask " : simulink/Logic and Bit Operations/Bitwise Operator  logicop=AND  UseBitMask=on  BitMask=hex2dec('1ffffc00')  BitMaskRealWorld=Stored Integer
  Multiply : Product  Inputs=**
  SDI : Constant  Value=2  OutDataTypeStr=uint32
  SSM : Constant  Value=3  OutDataTypeStr=uint32
  Scale : Constant  Value=1024  OutDataTypeStr=double
  Shift to SDI slot : ArithShift  BitShiftNumber=-8
  Shift to SSM slot : ArithShift  BitShiftNumber=-29
  Out1 : Outport
  wires:
  Data Type Conversion1/1 -> Out1/1
  Bitwise Operator/1 -> Display/1, Data Type Conversion1/1
  Label/1 -> Bitwise Operator/4
  Shift to SDI slot/1 -> Bitwise Operator/3
  Shift to SSM slot/1 -> Bitwise Operator/2
  SDI/1 -> Shift to SDI slot/1
  SSM/1 -> Shift to SSM slot/1
  "Mask "/1 -> Bitwise Operator/1
  Data Type Conversion/1 -> "Mask "/1
  Multiply/1 -> Data Type Conversion/1
  Divide/1 -> Multiply/1
  'shift' the double value 27 bits left/1 -> Multiply/2
  Scale/1 -> Divide/2
  In1/1 -> Divide/1

== system speedgoat_test_SN5659_R2021b/IO682/Encode Channel 7/Prepare RAW value ==
  note: The scale factor is
      | defined by the label
      | for this message.
  note: Manually construct the ARINC word.
      | This sample constructs a BNR format
      | word, but the data part could be
      | constructed from multiple data pieces
      | and discrete bits if the label requires it.
  note: Data
  note: The output has to be cast to a double
      | for input to the ARINC Encode block.
  In1 : Inport
  'shift' the double value 27 bits left : Constant  Value=2^28  OutDataTypeStr=double
  Bitwise Operator : simulink/Logic and Bit Operations/Bitwise Operator  logicop=OR  UseBitMask=off  NumInputPorts=4  BitMask=bin2dec('11011001')  BitMaskRealWorld=Stored Integer
  Data Type Conversion : DataTypeConversion  OutDataTypeStr=uint32
  Data Type Conversion1 : DataTypeConversion  OutDataTypeStr=double
  Display : Display
      settings: Format=hex (Stored Integer)
  Divide : Product  Inputs=*/
  Label : Constant  Value=base2dec( '103', 8 )  OutDataTypeStr=uint32
  "Mask " : simulink/Logic and Bit Operations/Bitwise Operator  logicop=AND  UseBitMask=on  BitMask=hex2dec('1ffffc00')  BitMaskRealWorld=Stored Integer
  Multiply : Product  Inputs=**
  SDI : Constant  Value=2  OutDataTypeStr=uint32
  SSM : Constant  Value=3  OutDataTypeStr=uint32
  Scale : Constant  Value=1024  OutDataTypeStr=double
  Shift to SDI slot : ArithShift  BitShiftNumber=-8
  Shift to SSM slot : ArithShift  BitShiftNumber=-29
  Out1 : Outport
  wires:
  In1/1 -> Divide/1
  Scale/1 -> Divide/2
  'shift' the double value 27 bits left/1 -> Multiply/2
  Divide/1 -> Multiply/1
  Multiply/1 -> Data Type Conversion/1
  Data Type Conversion/1 -> "Mask "/1
  "Mask "/1 -> Bitwise Operator/1
  SSM/1 -> Shift to SSM slot/1
  SDI/1 -> Shift to SDI slot/1
  Shift to SSM slot/1 -> Bitwise Operator/2
  Shift to SDI slot/1 -> Bitwise Operator/3
  Label/1 -> Bitwise Operator/4
  Bitwise Operator/1 -> Data Type Conversion1/1, Display/1
  Data Type Conversion1/1 -> Out1/1

== system speedgoat_test_SN5659_R2021b/IO682/Encode Channel 8/Prepare RAW value ==
  note: The output has to be cast to a double
      | for input to the ARINC Encode block.
  note: Data
  note: Manually construct the ARINC word.
      | This sample constructs a BNR format
      | word, but the data part could be
      | constructed from multiple data pieces
      | and discrete bits if the label requires it.
  note: The scale factor is
      | defined by the label
      | for this message.
  In1 : Inport
  'shift' the double value 27 bits left : Constant  Value=2^28  OutDataTypeStr=double
  Bitwise Operator : simulink/Logic and Bit Operations/Bitwise Operator  logicop=OR  UseBitMask=off  NumInputPorts=4  BitMask=bin2dec('11011001')  BitMaskRealWorld=Stored Integer
  Data Type Conversion : DataTypeConversion  OutDataTypeStr=uint32
  Data Type Conversion1 : DataTypeConversion  OutDataTypeStr=double
  Display : Display
      settings: Format=hex (Stored Integer)
  Divide : Product  Inputs=*/
  Label : Constant  Value=base2dec( '103', 8 )  OutDataTypeStr=uint32
  "Mask " : simulink/Logic and Bit Operations/Bitwise Operator  logicop=AND  UseBitMask=on  BitMask=hex2dec('1ffffc00')  BitMaskRealWorld=Stored Integer
  Multiply : Product  Inputs=**
  SDI : Constant  Value=2  OutDataTypeStr=uint32
  SSM : Constant  Value=3  OutDataTypeStr=uint32
  Scale : Constant  Value=1024  OutDataTypeStr=double
  Shift to SDI slot : ArithShift  BitShiftNumber=-8
  Shift to SSM slot : ArithShift  BitShiftNumber=-29
  Out1 : Outport
  wires:
  Data Type Conversion1/1 -> Out1/1
  Bitwise Operator/1 -> Display/1, Data Type Conversion1/1
  Label/1 -> Bitwise Operator/4
  Shift to SDI slot/1 -> Bitwise Operator/3
  Shift to SSM slot/1 -> Bitwise Operator/2
  SDI/1 -> Shift to SDI slot/1
  SSM/1 -> Shift to SSM slot/1
  "Mask "/1 -> Bitwise Operator/1
  Data Type Conversion/1 -> "Mask "/1
  Multiply/1 -> Data Type Conversion/1
  Divide/1 -> Multiply/1
  'shift' the double value 27 bits left/1 -> Multiply/2
  Scale/1 -> Divide/2
  In1/1 -> Divide/1
